simulink model "Single_Phase_FullWave_Full_Bridge_Rectifier"  (R2021a)
settings: Solver=VariableStepAuto  StartTime=0.0  StopTime=0.1  RelTol=1e-3
undefined symbols (not defined in the file): Ts
libraries: spsSeriesRLCBranchLib x4, spsDiodeLib x4, spsVoltageMeasurementLib x4, spsCurrentMeasurementLib x2, spsPowerLib x1, spsACVoltageSourceLib x1, spspowerguiLib x1
settings Model: Creator=EREN-PC  LastModifiedBy=EREN-PC
settings DataIOCC: ReturnWorkspaceOutputs=off

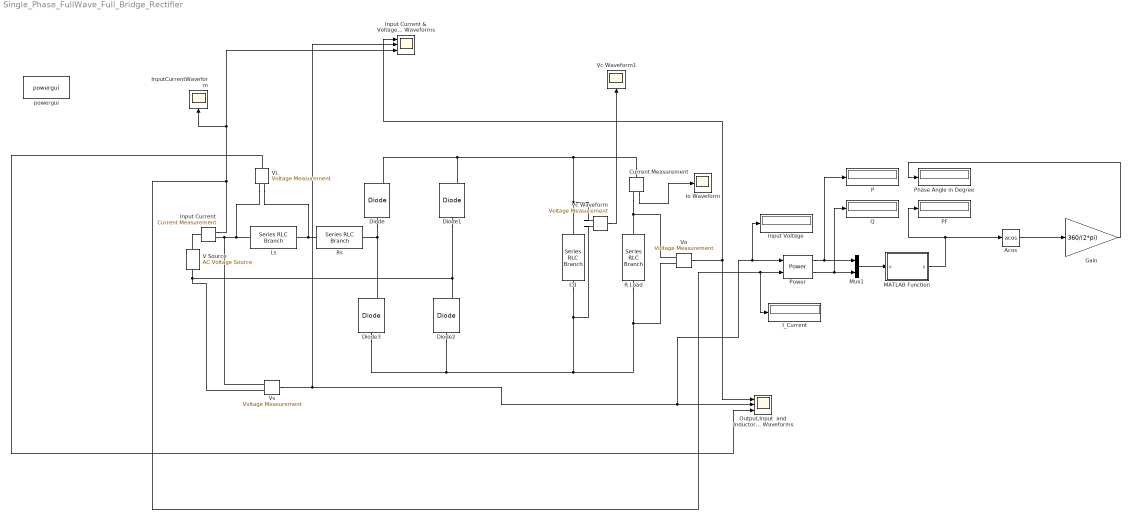
== system Single_Phase_FullWave_Full_Bridge_Rectifier ==
  Acos : Trigonometry  Operator=acos
  Cd : spsSeriesRLCBranchLib/Series RLC Branch  LConnTagsString=__new0  RConnTagsString=__new0  BranchType=C  Resistance=1  Inductance=1e-3  SetiL0=off  InitialCurrent=0  Capacitance=42e-3  Setx0=off  InitialVoltage=0  Measurements=None
  Current Measurement : spsCurrentMeasurementLib/Current Measurement  PhasorSimulation=off  OutputType=Complex  PSBequivalent=0
  Diode{,1..3} (4 alike) : spsDiodeLib/Diode  Ron=0.001  Lon=0  Vf=0.8  IC=0  UseSnubber=0  Rs=500  Cs=250e-9  Measurements=on
  Gain : Gain  Gain=360/(2*pi)
  I_Current : Display
  Input Current : spsCurrentMeasurementLib/Current Measurement  PhasorSimulation=off  OutputType=Complex  PSBequivalent=0
  "Input Current & Voltage , Output Voltage Waveforms" : Scope  NumInputPorts=3
  Input Voltage : Display
  InputCurrentWaveform : Scope
  Io Waveform : Scope
  Ls : spsSeriesRLCBranchLib/Series RLC Branch  LConnTagsString=__new0  RConnTagsString=__new0  BranchType=L  Resistance=1  Inductance=1e-3  SetiL0=off  InitialCurrent=0  Capacitance=1e-6  Setx0=off  InitialVoltage=0  Measurements=None
  MATLAB Function : MATLAB Function  TreatAsAtomicUnit=on
  Mux1 : Mux  Inputs=2
  Output,Input  and Inductor Voltage Waveforms : Scope  NumInputPorts=3
  P : Display
  PF : Display
  Phase Angle in Degree : Display
  Power : spsPowerLib/Power  Freq=50  Vinit=[230*sqrt(2) 0]  Iinit=[2, -54]  Ts=Ts
      settings: SourceProductBaseCode=PS
  Q : Display
  R Load : spsSeriesRLCBranchLib/Series RLC Branch  LConnTagsString=__new0  RConnTagsString=__new0  BranchType=R  Resistance=100  Inductance=1e-3  SetiL0=off  InitialCurrent=0  Capacitance=1e-6  Setx0=off  InitialVoltage=0  Measurements=None
  Rs : spsSeriesRLCBranchLib/Series RLC Branch  LConnTagsString=__new0  RConnTagsString=__new0  BranchType=R  Resistance=1e-3  Inductance=1e-3  SetiL0=off  InitialCurrent=0  Capacitance=1e-6  Setx0=off  InitialVoltage=0  Measurements=None
  V Source : spsACVoltageSourceLib/AC Voltage Source  Amplitude=325  Phase=0  Frequency=50  SampleTime=Ts  Measurements=Voltage  BusType=swing  Pref=10e3  Qref=0  Qmin=-inf  Qmax=+inf
  VL : spsVoltageMeasurementLib/Voltage Measurement  PhasorSimulation=off  OutputType=Complex  PSBequivalent=0
  Vc Waveform : spsVoltageMeasurementLib/Voltage Measurement  PhasorSimulation=off  OutputType=Complex  PSBequivalent=0
  Vc Waveform1 : Scope
  Vo : spsVoltageMeasurementLib/Voltage Measurement  PhasorSimulation=off  OutputType=Complex  PSBequivalent=0
  Vs : spsVoltageMeasurementLib/Voltage Measurement  PhasorSimulation=off  OutputType=Complex  PSBequivalent=0
  powergui : spspowerguiLib/powergui  Priority=1  SimulationMode=Discrete  SampleTime=1e-6  frequency=60  Iterations=50  frequencyindice=50  Pbase=100e6  ErrMax=1e-4  UnitsV=kV  UnitsW=MW  buscounter=0  FunctionMessages=off  echomessages=off  EnableUseOfTLC=off  CurrentSourceSwitches=off  DisableSnubberDevices=off  DisableRonSwitches=off  DisableVfSwitches=off  DisplayEquations=off  AutomaticDiscreteSolvers=off  SolverType=Tustin/Backward Euler (TBE)  Interpol=off  ExternalGateDelay=off  methode=off  Ts=100  x0status=blocks  SPID=on  SwTol=0  HookPort=off  NonlinearTolerance=1e-4  nMaxIteration=100  ContinueOnMaxIteration=off  RestoreLinks=warning  ResistiveCurrentMeasurement=off  Frange=[0:2:500]  Ylog=off  Xlog=on  ShowGrid=off  save=off  variable=ZData  structure=0  ZoomFFT=off  StartTime=0.0  cycles=1  DisplayStyle=1  fundamental=60  FreqAxis=off  MaxFrequency=1000  frequencyindicesteady=1  RmsSteady=1  display=off
  wires:
  Vo/1 -> Output,Input  and Inductor Voltage Waveforms/1, "Input Current & Voltage , Output Voltage Waveforms"/1
  Vs/1 -> Input Voltage/1, Power/1, Output,Input  and Inductor Voltage Waveforms/2, "Input Current & Voltage , Output Voltage Waveforms"/2
  VL/1 -> Output,Input  and Inductor Voltage Waveforms/3
  Current Measurement/1 -> Io Waveform/1
  Vc Waveform/1 -> Vc Waveform1/1
  Power/1 -> P/1, Mux1/1
  Power/2 -> Q/1, Mux1/2
  Mux1/1 -> MATLAB Function/1(u)
  MATLAB Function/1(y) -> Acos/1, PF/1
  Input Current/1 -> I_Current/1, Power/2, InputCurrentWaveform/1, "Input Current & Voltage , Output Voltage Waveforms"/3
  Acos/1 -> Gain/1
  Gain/1 -> Phase Angle in Degree/1
  connections:
  Vs/LConn1 -- Ls/LConn1 -- VL/LConn1 -- Input Current/RConn1
  Diode/LConn1 -- Rs/RConn1 -- Diode3/RConn1
  V Source/LConn1 -- Diode1/LConn1 -- Diode2/RConn1 -- Vs/LConn2
  Diode/RConn1 -- Diode1/RConn1 -- Current Measurement/LConn1 -- Vc Waveform/LConn1 -- Cd/LConn1
  R Load/RConn1 -- Vc Waveform/LConn2 -- Cd/RConn1 -- Diode2/LConn1 -- Diode3/LConn1 -- Vo/LConn2
  Rs/LConn1 -- VL/LConn2 -- Ls/RConn1
  Vo/LConn1 -- R Load/LConn1 -- Current Measurement/RConn1
  Input Current/LConn1 -- V Source/RConn1

== matlab function Single_Phase_FullWave_Full_Bridge_Rectifier/MATLAB Function ==
  data: u input; y output
function y = fcn(u)

y = u(1)/(sqrt((u(1)*u(1))+u(2)*u(2)));
